simulink model "design_project_openloop_linear_bk_1"  (R2023b)
settings: Solver=VariableStepAuto  StartTime=0.0  StopTime=500  RelTol=1e-3
settings Model: Creator=qingyu  LastModifiedBy=qingyu

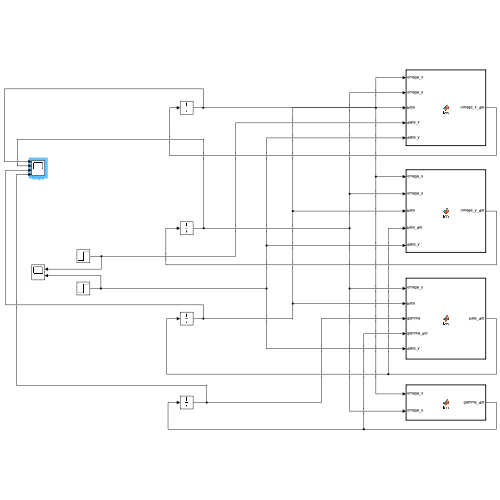
[thumbnail: Simulink's stored preview of the top-level diagram]
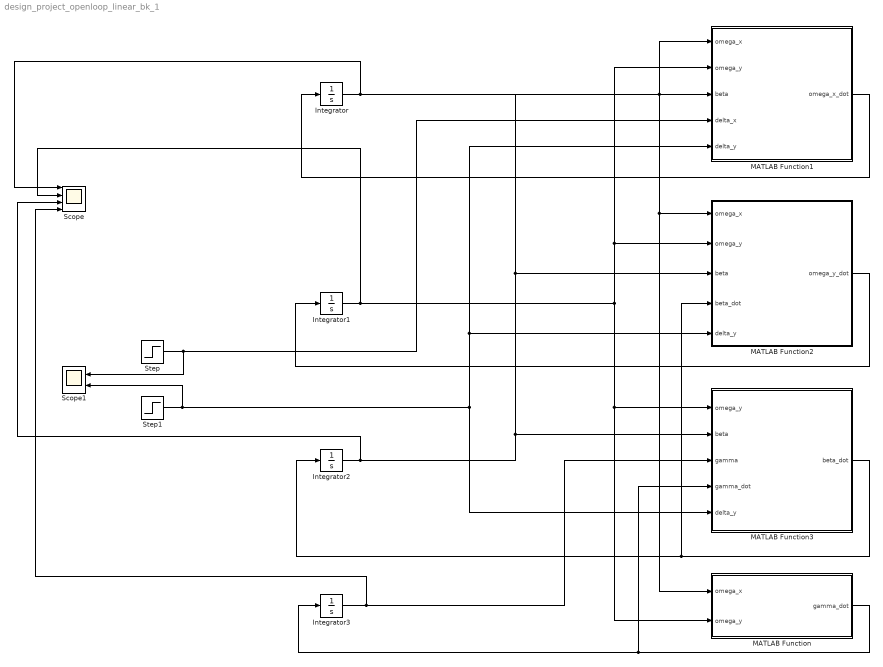
== system design_project_openloop_linear_bk_1 ==
  Integrator : Integrator  InitialCondition=0.1
  Integrator1 : Integrator  InitialCondition=0.1
  Integrator2 : Integrator  InitialCondition=0.05
  Integrator3 : Integrator  InitialCondition=0.05
  MATLAB Function : MATLAB Function  TreatAsAtomicUnit=on
  MATLAB Function1 : MATLAB Function  TreatAsAtomicUnit=on
  MATLAB Function2 : MATLAB Function  TreatAsAtomicUnit=on
  MATLAB Function3 : MATLAB Function  TreatAsAtomicUnit=on
  Scope : Scope  NumInputPorts=4
  Scope1 : Scope  NumInputPorts=2
  Step : Step  After=0  SampleTime=0
  Step1 : Step  After=0.01  SampleTime=0
  wires:
  Integrator/1 -> MATLAB Function/1(omega_x), MATLAB Function2/1(omega_x), MATLAB Function1/1(omega_x), Scope/1
  Integrator1/1 -> MATLAB Function/2(omega_y), MATLAB Function3/1(omega_y), MATLAB Function1/2(omega_y), MATLAB Function2/2(omega_y), Scope/2
  Integrator2/1 -> MATLAB Function2/3(beta), MATLAB Function1/3(beta), MATLAB Function3/2(beta), Scope/3
  Integrator3/1 -> MATLAB Function3/3(gamma), Scope/4
  Step/1 -> Scope1/1, MATLAB Function1/4(delta_x)
  Step1/1 -> Scope1/2, MATLAB Function1/5(delta_y), MATLAB Function2/5(delta_y), MATLAB Function3/5(delta_y)
  MATLAB Function1/1(omega_x_dot) -> Integrator/1
  MATLAB Function2/1(omega_y_dot) -> Integrator1/1
  MATLAB Function3/1(beta_dot) -> Integrator2/1, MATLAB Function2/4(beta_dot)
  MATLAB Function/1(gamma_dot) -> Integrator3/1, MATLAB Function3/4(gamma_dot)

== matlab function design_project_openloop_linear_bk_1/MATLAB Function1 ==
  data: omega_x input; omega_x_dot output; omega_y input; beta input; delta_x input; delta_y input

function omega_x_dot = fcn(omega_x, omega_y, beta, delta_x, delta_y)

b11 = 1.8600;
b12 = 0.6600;
b14 = 8.8000;
b17 = 0.7800;
b18 = 0.9800;

omega_x_dot = 0;
omega_x_dot = omega_x_dot - b11*omega_x;
omega_x_dot = omega_x_dot - b12*omega_y;
omega_x_dot = omega_x_dot - b14*beta;
omega_x_dot = omega_x_dot - b18*delta_x;
omega_x_dot = omega_x_dot - b17*delta_y;

== matlab function design_project_openloop_linear_bk_1/MATLAB Function ==
  data: omega_x input; gamma_dot output; omega_y input
function gamma_dot = fcn(omega_x,omega_y)

b52 = -0.0034;

gamma_dot = 0;
gamma_dot = gamma_dot + omega_x;
gamma_dot = gamma_dot + b52*omega_y;

== matlab function design_project_openloop_linear_bk_1/MATLAB Function2 ==
  data: omega_x input; omega_y_dot output; omega_y input; beta input; beta_dot input; delta_y input
function omega_y_dot = fcn(omega_x,omega_y,beta,beta_dot,delta_y)

b21 = 0.0200;
b22 = 0.2000;
b24 = 3.0000;
b24_dot = 0;
b27 = 0.9000;

omega_y_dot = 0;
omega_y_dot = omega_y_dot - b21*omega_x;
omega_y_dot = omega_y_dot - b22*omega_y;
omega_y_dot = omega_y_dot - b24*beta;
omega_y_dot = omega_y_dot - b24_dot*beta_dot;
omega_y_dot = omega_y_dot - b27*delta_y;

== matlab function design_project_openloop_linear_bk_1/MATLAB Function3 ==
  data: omega_y input; beta input; gamma input; beta_dot output; gamma_dot input; delta_y input
function beta_dot = fcn(omega_y, beta, gamma, gamma_dot, delta_y)

b32     = -1;
b34     =  0.0600;
b35     = -0.0280;
b37     =  0.0180;
a33     = -3.3600e-05;
alpha   =  0.2618;

beta_dot = 0;
beta_dot = beta_dot - b32*omega_y;
beta_dot = beta_dot - (b34+a33)*beta;
beta_dot = beta_dot - b35*gamma;
beta_dot = beta_dot + alpha*gamma_dot;
beta_dot = beta_dot - b37*delta_y;
